simulink model "slm_paper"  (Simulink 8.6)
settings: Solver=ode45  StartTime=0.0  StopTime=30  RelTol=1e-3
libraries: mblibv1 x12, simulink x3, aerolibconvert2 x2
settings Model: Creator=debraj  LastModifiedBy=Ayansengupta17
settings SolverCC: ZeroCrossControl=DisableAll
settings DebuggingCC: FcnCallInpInsideContextMsg=UseLocalSettings
settings ConfigComp: CovSFcnEnable=off
settings SimMechanicsCC: VisOnUpdateDiagram=on  VisDuringSimulation=on
settings ConfigurationSet: Description=SimMechanics 2G

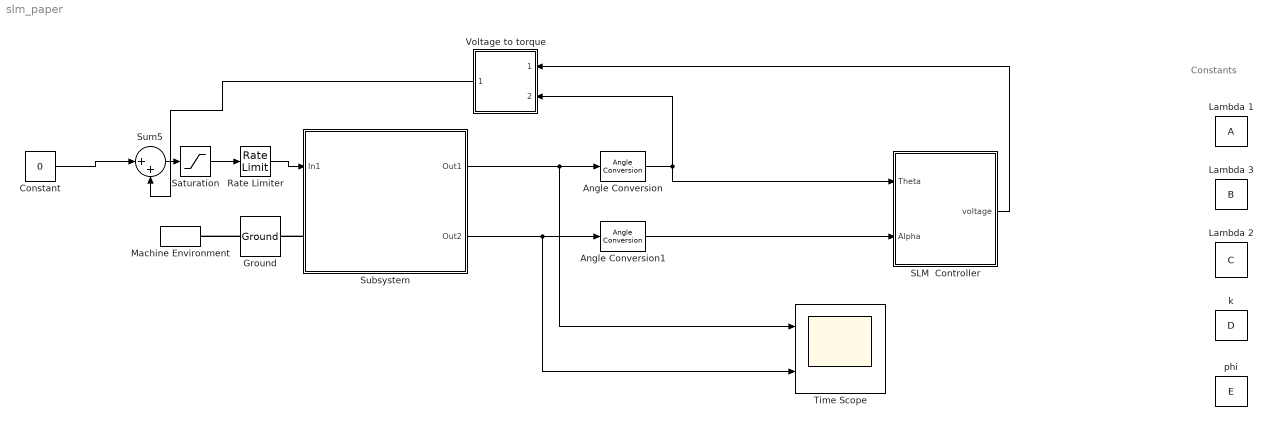
== system slm_paper ==
  note: Constants
  Angle Conversion : aerolibconvert2/Angle Conversion  IU=deg  OU=rad
  Angle Conversion1 : aerolibconvert2/Angle Conversion  IU=deg  OU=rad
  Constant : Constant  Value=0
  Ground : mblibv1/Bodies/Ground  UpdateFromCAD=off  LeftPortType=env  RightPortType=workingframe  PhysicalDomain=Mechanical  DialogClass=GroundBlock  CoordPosition=[0 0 0]  CoordPositionUnits=m  StateVectorMgrId=0  MachineId=[1 0]  ShowEnvPort=on  ParameterChecksum=[2459669987, 3834972678, 64255769, 951891124]  TopologyChecksum=[3132375730, 187115475, 220121263, 2848747769]
  Lambda 1 : DataStoreMemory  ReadBeforeWriteMsg=warning  WriteAfterWriteMsg=warning  WriteAfterReadMsg=warning  InitialValue=0.2
  Lambda 2 : DataStoreMemory  DataStoreName=C  ReadBeforeWriteMsg=warning  WriteAfterWriteMsg=warning  WriteAfterReadMsg=warning  InitialValue=0.9
  Lambda 3 : DataStoreMemory  DataStoreName=B  ReadBeforeWriteMsg=warning  WriteAfterWriteMsg=warning  WriteAfterReadMsg=warning  InitialValue=1
  Machine Environment : mblibv1/Bodies/Machine Environment  Tag=Factory ground  PortType=env  PhysicalDomain=Mechanical  DialogTemplateClass=MECH.MachineEnvironment  SyncWhenCopied=off  Gravity=[0 0 -9.81]  GravityUnits=m/s^2  GravityAsSignal=off  Dimensionality=Auto-detect  AnalysisType=Forward dynamics  LinearAssemblyTolerance=1e-3  LinearAssemblyToleranceUnits=m  AngularAssemblyTolerance=1e-3  AngularAssemblyToleranceUnits=rad  ConstraintSolverType=Stabilizing  ConstraintRelTolerance=1e-4  ConstraintAbsTolerance=1e-4  UseRobustSingularityHandling=off  RedundancyAnalysisToleranceType=Automatically select tolerance  RedundancyAnalysisTolerance=1e-14  StatePerturbationType=Fixed  PerturbationSize=1e-5  VisualizeMachine=on  BodyVisualizationType=Use model default body geometries  BodyColorSelMode=Use model default  DefaultBodyColor=[1 0 0]
  Rate Limiter : RateLimiter
  SLM  Controller : Subsystem
  Saturation : Saturate  UpperLimit=200  LowerLimit=-200  ZeroCross=off
  Subsystem : Subsystem
      mask init:
      | throttle = imread('spe_mech_invpend.jpg');
      mask Display: image(throttle)
  Sum5 : Sum  Inputs=|++
  Time Scope : Scope  NumInputPorts=2
  "Voltage to torque " : Subsystem
  k : DataStoreMemory  DataStoreName=D  ReadBeforeWriteMsg=warning  WriteAfterWriteMsg=warning  WriteAfterReadMsg=warning  InitialValue=9
  phi : DataStoreMemory  DataStoreName=E  ReadBeforeWriteMsg=warning  WriteAfterWriteMsg=warning  WriteAfterReadMsg=warning  InitialValue=0.5
  wires:
  Subsystem/2(Out2) -> Time Scope/2, Angle Conversion1/1
  Saturation/1 -> Rate Limiter/1
  Rate Limiter/1 -> Subsystem/1(In1)
  Sum5/1 -> Saturation/1
  Constant/1 -> Sum5/1
  Subsystem/1(Out1) -> Time Scope/1, Angle Conversion/1
  Angle Conversion/1 -> SLM  Controller/1(Theta), "Voltage to torque "/2(Theta)
  "Voltage to torque "/1("Torque ") -> Sum5/2
  Angle Conversion1/1 -> SLM  Controller/2("Alpha ")
  SLM  Controller/1("voltage ") -> "Voltage to torque "/1(voltage)
  connections:
  Ground/LConn1 -- Machine Environment/RConn1
  Subsystem/LConn1 -- Ground/RConn1

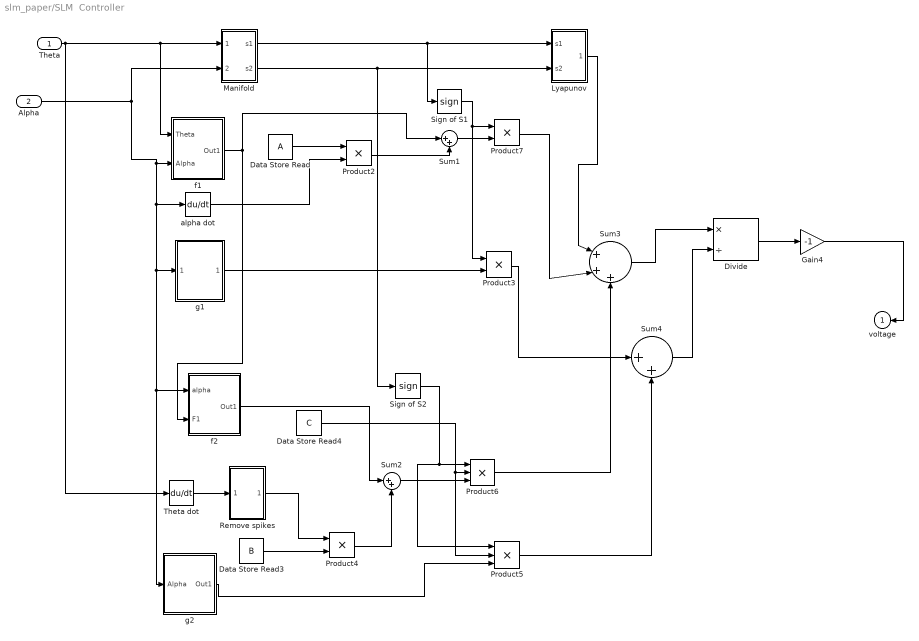
== system slm_paper/SLM  Controller ==
  Theta : Inport
  "Alpha " : Inport  Port=2
  Data Store Read : DataStoreRead
  Data Store Read3 : DataStoreRead  DataStoreName=B
  Data Store Read4 : DataStoreRead  DataStoreName=C
  Divide : Product  Inputs=*/
  Gain4 : Gain  Gain=-1
  "Lyapunov " : Subsystem
  Manifold : Subsystem
  Product{2..4,7} (4 alike) : Product
  Product5 : Product  Inputs=3
  Product6 : Product  Inputs=3
  Remove spikes : Subsystem
  Sign of S1 : Signum  ZeroCross=off
  Sign of S2 : Signum  ZeroCross=off
  Sum1 : Sum  Inputs=|++
  Sum2 : Sum  Inputs=|++
  Sum3 : Sum  Inputs=|+++
  Sum4 : Sum  Inputs=|++
  Theta dot : Derivative
  "alpha dot " : Derivative  CoefficientInTFapproximation=0.00001
  f1 : Subsystem
  f2 : Subsystem
  g1 : Subsystem
  g2 : Subsystem
  "voltage " : Outport
  wires:
  Product2/1 -> Sum1/2
  Sign of S1/1 -> Product3/1, Product7/1
  Sum1/1 -> Product7/2
  Sign of S2/1 -> Product6/1, Product5/1
  Sum2/1 -> Product6/3
  Product3/1 -> Sum4/1
  Manifold/1(s1) -> Sign of S1/1, "Lyapunov "/1(s1)
  Divide/1 -> Gain4/1
  Theta dot/1 -> Remove spikes/1(In1)
  "Lyapunov "/1(Out1) -> Sum3/1
  f2/1(Out1) -> Sum2/1
  Product5/1 -> Sum4/2
  Product4/1 -> Sum2/2
  Sum3/1 -> Divide/1
  Manifold/2(s2) -> Sign of S2/1, "Lyapunov "/2(s2)
  f1/1(Out1) -> Sum1/1, f2/2("F1 ")
  Sum4/1 -> Divide/2
  g2/1(Out1) -> Product5/3
  Data Store Read4/1 -> Product5/2, Product6/2
  Product7/1 -> Sum3/2
  Product6/1 -> Sum3/3
  "alpha dot "/1 -> Product2/2
  "Alpha "/1 -> Manifold/2("alpha "), "alpha dot "/1, f2/1(alpha), g2/1("Alpha "), g1/1("Alpha "), f1/2("Alpha ")
  Remove spikes/1(Out1) -> Product4/1
  Data Store Read3/1 -> Product4/2
  Gain4/1 -> "voltage "/1
  g1/1(Out1) -> Product3/2
  Data Store Read/1 -> Product2/1
  Theta/1 -> Theta dot/1, Manifold/1(theta), f1/1(Theta)

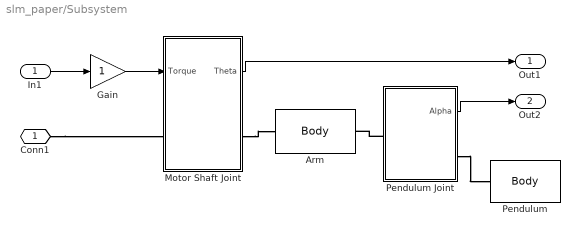
== system slm_paper/Subsystem ==
  In1 : Inport
  Arm : mblibv1/Bodies/Body  Tag=Factory generic  Description=Mechanical Blockset  LConnTagsString=CS1  RConnTagsString=CS2  UpdateFromCAD=off  DialogClass=MechanicalBodyBlock  Mass=0.028  MassUnits=kg  InertiaUnits=kg*m^2  Inertia=[0 0 0;0 0 0;0 0 0.000123]  Shape=Cylinder  ShapeDims=[1 1]  ShapeUnits=m  ShapeUse=false  Density=1  DensityUnits=kg/m^3  DensityUse=false  GraphicsMode=MACHINE_DEFAULT  BodyColorSelMode=MACHINE_DEFAULT  BodyColor=[1 0 0]  AttachedToCS=CG  CG=Left$CG$[0 0.08260/2 0]$CS1$CS1$m$[0 0 0]$Euler X-Y-Z$deg$WORLD$false$none  WorkingFrames=Left$CS1$[0 0 0]$WORLD$WORLD$m$[0 0 0]$Euler X-Y-Z$deg$WORLD$true$none#Right$CS2$[0 0.08260 0]$CS1$CS1$m$[0 0 0]$Euler X-Y-Z$deg$WORLD$true$none  CGPos=[0 0.08260/2 0]  CGRot=[0 0 0]  CS0Pos=[]  CS0Rot=[]  CS1Pos=[0 0 0]  CS1Rot=[0 0 0]  CS2Pos=[0 0.08260 0]  CS2Rot=[0 0 0]  CS3Pos=[]  CS3Rot=[]  CS4Pos=[]  CS4Rot=[]  CS5Pos=[]  CS5Rot=[]  CS6Pos=[]  CS6Rot=[]  CS7Pos=[]  CS7Rot=[]  CS8Pos=[]  CS8Rot=[]  CS9Pos=[]  CS9Rot=[]  CS10Pos=[]  CS10Rot=[]  CS11Pos=[]  CS11Rot=[]  CS12Pos=[]  CS12Rot=[]  CS13Pos=[]  CS13Rot=[]  CS14Pos=[]  CS14Rot=[]  CS15Pos=[]  CS15Rot=[]  CS16Pos=[]  CS16Rot=[]  CS17Pos=[]  CS17Rot=[]  CS18Pos=[]  CS18Rot=[]  CS19Pos=[]  CS19Rot=[]  CS20Pos=[]  CS20Rot=[]
  Gain : Gain
  Motor Shaft Joint : Subsystem
  Pendulum : mblibv1/Bodies/Body  Tag=Factory generic  Description=Mechanical Blockset  LConnTagsString=CS1  UpdateFromCAD=off  DialogClass=MechanicalBodyBlock  Mass=0.027  MassUnits=kg  InertiaUnits=kg*m^2  Inertia=[0 0 0;0 0 0;0 0 0.00011]  Shape=Cylinder  ShapeDims=[1 1]  ShapeUnits=m  ShapeUse=false  Density=1  DensityUnits=kg/m^3  DensityUse=false  GraphicsMode=MACHINE_DEFAULT  BodyColorSelMode=MACHINE_DEFAULT  BodyColor=[1 0 0]  AttachedToCS=CG  CG=Left$CG$[0 0 0.191/2]$CS1$CS1$m$[0 0 0]$Euler X-Y-Z$deg$WORLD$false$none  WorkingFrames=Left$CS1$[0 0 0]$ADJOINING$ADJOINING$m$[0 0 0]$Euler X-Y-Z$deg$WORLD$true$none#Right$CS2$[0 0 0.191]$CS1$CS1$m$[0 0 0]$Euler X-Y-Z$deg$WORLD$false$none  CGPos=[0 0 0.191/2]  CGRot=[0 0 0]  CS0Pos=[]  CS0Rot=[]  CS1Pos=[0 0 0]  CS1Rot=[0 0 0]  CS2Pos=[0 0 0.191]  CS2Rot=[0 0 0]  CS3Pos=[]  CS3Rot=[]  CS4Pos=[]  CS4Rot=[]  CS5Pos=[]  CS5Rot=[]  CS6Pos=[]  CS6Rot=[]  CS7Pos=[]  CS7Rot=[]  CS8Pos=[]  CS8Rot=[]  CS9Pos=[]  CS9Rot=[]  CS10Pos=[]  CS10Rot=[]  CS11Pos=[]  CS11Rot=[]  CS12Pos=[]  CS12Rot=[]  CS13Pos=[]  CS13Rot=[]  CS14Pos=[]  CS14Rot=[]  CS15Pos=[]  CS15Rot=[]  CS16Pos=[]  CS16Rot=[]  CS17Pos=[]  CS17Rot=[]  CS18Pos=[]  CS18Rot=[]  CS19Pos=[]  CS19Rot=[]  CS20Pos=[]  CS20Rot=[]
  Pendulum Joint : Subsystem
  Conn1 : PMIOPort  Port=1  Side=Left
  Out1 : Outport
  Out2 : Outport  Port=2
  wires:
  Motor Shaft Joint/1(Theta) -> Out1/1
  In1/1 -> Gain/1
  Pendulum Joint/1(Alpha) -> Out2/1
  Gain/1 -> Motor Shaft Joint/1(Torque)
  connections:
  Motor Shaft Joint/RConn1 -- Arm/LConn1
  Pendulum Joint/LConn1 -- Arm/RConn1
  Pendulum Joint/RConn1 -- Pendulum/LConn1
  Conn1/RConn1 -- Motor Shaft Joint/LConn1

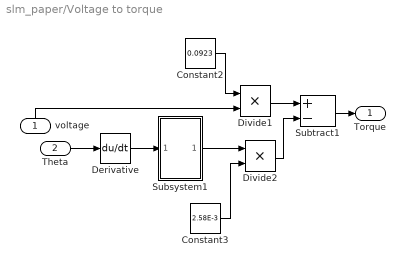
== system slm_paper/Voltage to torque  ==
  voltage : Inport
  Theta : Inport  Port=2
  Constant2 : Constant  Value=0.0923
  Constant3 : Constant  Value=2.58E-3
  Derivative : Derivative  CoefficientInTFapproximation=0.00001
  Divide1 : Product  Inputs=**
  Divide2 : Product  Inputs=**
  Subsystem1 : Subsystem
  Subtract1 : Sum  Inputs=+-
  "Torque " : Outport
  wires:
  Constant2/1 -> Divide1/1
  Subtract1/1 -> "Torque "/1
  Divide2/1 -> Subtract1/2
  Divide1/1 -> Subtract1/1
  voltage/1 -> Divide1/2
  Constant3/1 -> Divide2/2
  Theta/1 -> Derivative/1
  Derivative/1 -> Subsystem1/1(In1)
  Subsystem1/1(Out1) -> Divide2/1

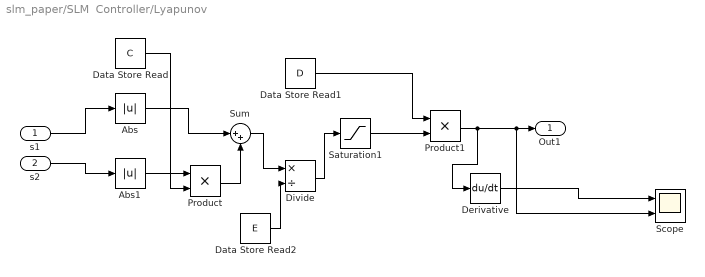
== system slm_paper/SLM  Controller/Lyapunov  ==
  s1 : Inport
  s2 : Inport  Port=2
  Abs : Abs
  Abs1 : Abs
  Data Store Read : DataStoreRead  DataStoreName=C
  Data Store Read1 : DataStoreRead  DataStoreName=D
  Data Store Read2 : DataStoreRead  DataStoreName=E
  Derivative : Derivative
  Divide : Product  Inputs=*/
  Product : Product
  Product1 : Product
  Saturation1 : Saturate  UpperLimit=1  LowerLimit=-1  ZeroCross=off
  Scope : Scope  NumInputPorts=2
  Sum : Sum  Inputs=|++
  Out1 : Outport
  wires:
  Data Store Read/1 -> Product/2
  s2/1 -> Abs1/1
  s1/1 -> Abs/1
  Abs1/1 -> Product/1
  Abs/1 -> Sum/1
  Product/1 -> Sum/2
  Saturation1/1 -> Product1/2
  Data Store Read1/1 -> Product1/1
  Sum/1 -> Divide/1
  Divide/1 -> Saturation1/1
  Data Store Read2/1 -> Divide/2
  Product1/1 -> Derivative/1, Scope/2, Out1/1
  Derivative/1 -> Scope/1

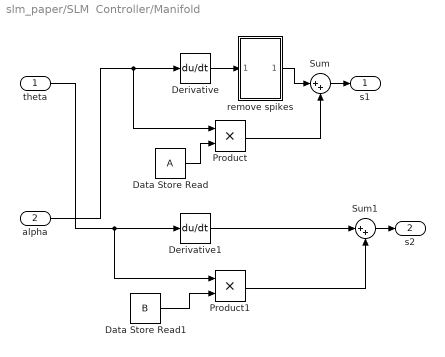
== system slm_paper/SLM  Controller/Manifold ==
  theta : Inport
  "alpha " : Inport  Port=2
  Data Store Read : DataStoreRead
  Data Store Read1 : DataStoreRead  DataStoreName=B
  Derivative : Derivative
  Derivative1 : Derivative
  Product : Product
  Product1 : Product
  Sum : Sum  Inputs=|++
  Sum1 : Sum  Inputs=|++
  "remove spikes " : Subsystem
  s1 : Outport
  s2 : Outport  Port=2
  wires:
  Sum/1 -> s1/1
  Sum1/1 -> s2/1
  Product/1 -> Sum/2
  Product1/1 -> Sum1/2
  Data Store Read/1 -> Product/2
  Data Store Read1/1 -> Product1/2
  Derivative1/1 -> Sum1/1
  Derivative/1 -> "remove spikes "/1(In1)
  "remove spikes "/1(Out1) -> Sum/1
  "alpha "/1 -> Product/1, Derivative/1
  theta/1 -> Product1/1, Derivative1/1

== system slm_paper/SLM  Controller/Remove spikes ==
  In1 : Inport
  Compare To Constant : simulink/Logic and Bit Operations/Compare To Constant  relop=<=  const=50  OutDataTypeStr=boolean
  Product1 : Product
  Out1 : Outport
  wires:
  In1/1 -> Product1/2, Compare To Constant/1
  Product1/1 -> Out1/1
  Compare To Constant/1 -> Product1/1

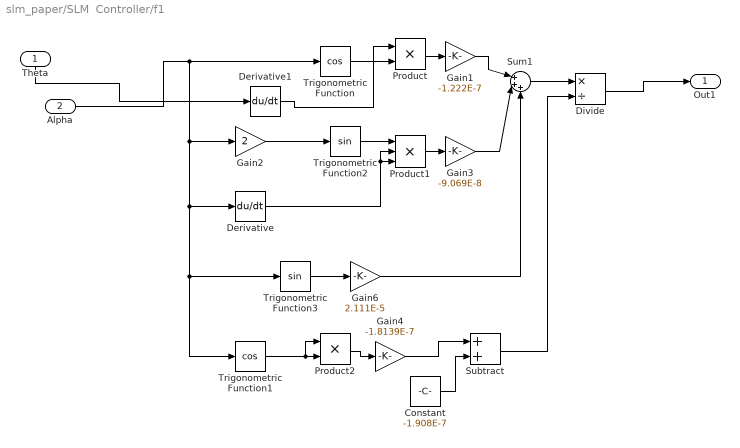
== system slm_paper/SLM  Controller/f1 ==
  Theta : Inport
  "Alpha " : Inport  Port=2
  Constant : Constant  Value=-1.908E-7
  Derivative : Derivative
  Derivative1 : Derivative
  Divide : Product  Inputs=*/
  Gain1 : Gain  Gain=-1.222E-7
  Gain2 : Gain  Gain=2
  Gain3 : Gain  Gain=-9.069E-8
  Gain4 : Gain  Gain=-1.8139E-7
  Gain6 : Gain  Gain=2.111E-5
  Product : Product
  Product1 : Product  Inputs=3
  Product2 : Product
  Subtract : Sum
  Sum1 : Sum  Inputs=|+++
  Trigonometric Function : Trigonometry  Operator=cos
  Trigonometric Function1 : Trigonometry  Operator=cos
  Trigonometric Function2 : Trigonometry
  Trigonometric Function3 : Trigonometry
  Out1 : Outport
  wires:
  Gain3/1 -> Sum1/2
  Trigonometric Function2/1 -> Product1/1
  Gain1/1 -> Sum1/1
  Trigonometric Function/1 -> Product/2
  Product1/1 -> Gain3/1
  Gain2/1 -> Trigonometric Function2/1
  Product/1 -> Gain1/1
  Trigonometric Function1/1 -> Product2/1, Product2/2
  Product2/1 -> Gain4/1
  Gain4/1 -> Subtract/1
  Constant/1 -> Subtract/2
  Sum1/1 -> Divide/1
  Subtract/1 -> Divide/2
  Divide/1 -> Out1/1
  Derivative/1 -> Product1/3, Product1/2
  Derivative1/1 -> Product/1
  Trigonometric Function3/1 -> Gain6/1
  Gain6/1 -> Sum1/3
  "Alpha "/1 -> Trigonometric Function3/1, Trigonometric Function1/1, Derivative/1, Gain2/1, Trigonometric Function/1
  Theta/1 -> Derivative1/1

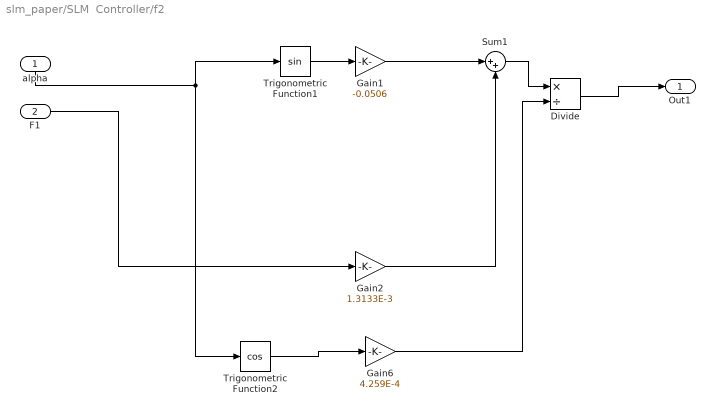
== system slm_paper/SLM  Controller/f2 ==
  alpha : Inport
  "F1 " : Inport  Port=2
  Divide : Product  Inputs=*/
  Gain1 : Gain  Gain=-0.0506
  Gain2 : Gain  Gain=1.3133E-3
  Gain6 : Gain  Gain=4.259E-4
  Sum1 : Sum  Inputs=|++
  Trigonometric Function1 : Trigonometry
  Trigonometric Function2 : Trigonometry  Operator=cos
  Out1 : Outport
  wires:
  "F1 "/1 -> Gain2/1
  alpha/1 -> Trigonometric Function1/1, Trigonometric Function2/1
  Sum1/1 -> Divide/1
  Divide/1 -> Out1/1
  Trigonometric Function2/1 -> Gain6/1
  Gain6/1 -> Divide/2
  Trigonometric Function1/1 -> Gain1/1
  Gain1/1 -> Sum1/1
  Gain2/1 -> Sum1/2

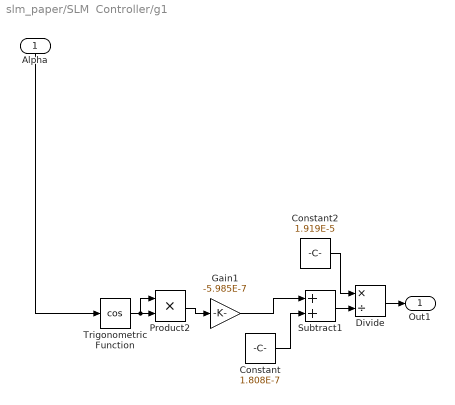
== system slm_paper/SLM  Controller/g1 ==
  "Alpha " : Inport
  Constant : Constant  Value=1.808E-7
  Constant2 : Constant  Value=1.919E-5
  Divide : Product  Inputs=*/
  Gain1 : Gain  Gain=-5.985E-7
  Product2 : Product
  Subtract1 : Sum
  Trigonometric Function : Trigonometry  Operator=cos
  Out1 : Outport
  wires:
  Subtract1/1 -> Divide/2
  Trigonometric Function/1 -> Product2/1, Product2/2
  Product2/1 -> Gain1/1
  Constant2/1 -> Divide/1
  "Alpha "/1 -> Trigonometric Function/1
  Divide/1 -> Out1/1
  Gain1/1 -> Subtract1/1
  Constant/1 -> Subtract1/2

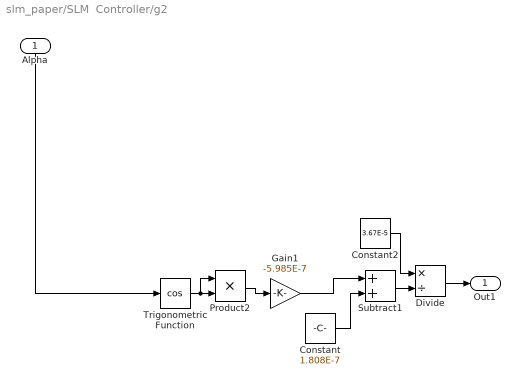
== system slm_paper/SLM  Controller/g2 ==
  "Alpha " : Inport
  Constant : Constant  Value=1.808E-7
  Constant2 : Constant  Value=3.67E-5
  Divide : Product  Inputs=*/
  Gain1 : Gain  Gain=-5.985E-7
  Product2 : Product
  Subtract1 : Sum
  Trigonometric Function : Trigonometry  Operator=cos
  Out1 : Outport
  wires:
  "Alpha "/1 -> Trigonometric Function/1
  Divide/1 -> Out1/1
  Subtract1/1 -> Divide/2
  Trigonometric Function/1 -> Product2/1, Product2/2
  Product2/1 -> Gain1/1
  Constant2/1 -> Divide/1
  Gain1/1 -> Subtract1/1
  Constant/1 -> Subtract1/2

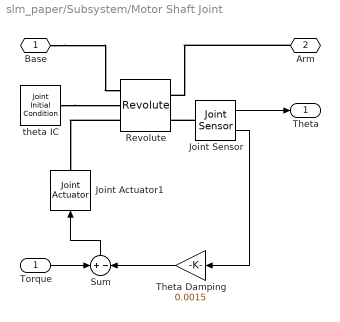
== system slm_paper/Subsystem/Motor Shaft Joint ==
  Torque : Inport
  Joint Actuator1 : mblibv1/Sensors &  Actuators/Joint Actuator  UpdateFromCAD=off  PhysicalDomain=Mechanical  PortType=blob  ActuationStyle=Force  AngleUnits=deg  ArcVelocityUnits=deg/s  ArcAccelerationUnits=deg/s^2  CoordPositionUnits=m  VelocityUnits=m/s  AccelerationUnits=m/s^2  ForceUnits=N  TorqueUnits=N-m  ActiveIO=on  Width=1  DialogClass=MechanicalActuatorBlock  Primitive=R1  ReferenceFrame=Absolute (World)
  Joint Sensor : mblibv1/Sensors &  Actuators/Joint Sensor  Description=Mechanical Blockset  UpdateFromCAD=off  PhysicalDomain=Mechanical  PortType=blob  Muxed=off  Pose=off  Angle=on  AngleUnits=deg  ArcVelocity=on  ArcVelocityUnits=rad/s  ArcAcceleration=off  ArcAccelerationUnits=deg/s^2  CoordPosition=on  CoordPositionUnits=m  Velocity=off  VelocityUnits=m/s  Acceleration=off  AccelerationUnits=m/s^2  Quaternion=on  QuaternionDT=off  QuaternionDDT=off  QuaternionUnits=off  OutputVector=[ 1 1 ]  ActiveIO=on  Width=2  DialogClass=MechanicalSensorBlock  Primitive=R1  Force=off  ForceUnits=N  Torque=off  TorqueUnits=N*m  ReferenceFrame=Absolute (INERTIAL)  ReactionSensedSide=Base  ReactionReferenceFrame=Absolute (World)  ReactionForce=off  ReactionForceUnits=N  ReactionMoment=off  ReactionMomentUnits=N*m
  Revolute : mblibv1/Joints/Revolute  Tag=Factory generic  Description=Mechanical Blockset  LConnTagsString=__newl0|SA1|SA2  RConnTagsString=__newr0|SA1  UpdateFromCAD=off  NumSAPorts=3  CutJoint=off  MarkAsCut=off  Primitives=revolute  PrimitiveProps=R1$Base$[0 0 1]$revolute  DialogClass=JointBlock  R1Axis=[0 0 1]
  Sum : Sum  Inputs=+|-  SaturateOnIntegerOverflow=on  InputSameDT=on  OutDataTypeStr=Inherit: Same as first input
  Theta Damping : Gain  Gain=0.0015  SaturateOnIntegerOverflow=on  OutDataTypeStr=Inherit: Same as input  ParamDataTypeStr=Inherit: Same as input
  theta IC : mblibv1/Sensors &  Actuators/Joint Initial Condition  Description=Mechanical Blockset  UpdateFromCAD=off  LeftPortType=blob  RightPortType=blob  PhysicalDomain=Mechanical  DialogClass=InitialConditionBlock  Primitive=R1  CoordPosition=0  Velocity=0.0  AngleUnits=deg  ArcVelocityUnits=deg/s  CoordPositionUnits=m  VelocityUnits=m/s  InitialConditions=P1$false$0$m$rad$0$m/s$rad/s#P2$false$0$m$rad$0$m/s$rad/s#P3$false$0$m$rad$0$m/s$rad/s#R1$true$0$m$deg$0.0$m/s$deg/s#R2$false$0$m$rad$0$m/s$rad/s#R3$false$0$m$rad$0$m/s$rad/s#S$false$0$m$rad$0$m/s$rad/s  P1PIC=0  P1VIC=0  P2PIC=0  P2VIC=0  P3PIC=0  P3VIC=0  R1PIC=0  R1VIC=0.0  R2PIC=0  R2VIC=0  R3PIC=0  R3VIC=0  SPIC=0  SVIC=0
  Base : PMIOPort  Port=1  Side=Left
  Arm : PMIOPort  Port=2  Side=Right
  Theta : Outport
  wires:
  Joint Sensor/2 -> Theta Damping/1
  Joint Sensor/1 -> Theta/1
  Torque/1 -> Sum/1
  Theta Damping/1 -> Sum/2
  Sum/1 -> Joint Actuator1/1
  connections:
  Joint Sensor/LConn1 -- Revolute/RConn2
  Revolute/LConn3 -- Joint Actuator1/RConn1
  theta IC/RConn1 -- Revolute/LConn2
  Arm/RConn1 -- Revolute/RConn1
  Base/RConn1 -- Revolute/LConn1

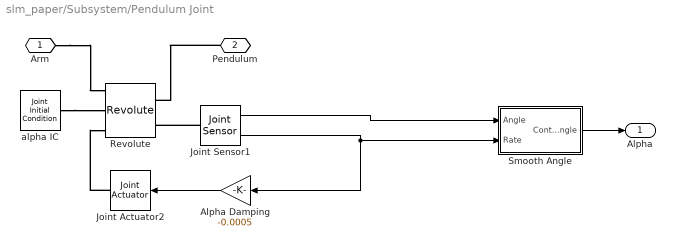
== system slm_paper/Subsystem/Pendulum Joint ==
  Alpha Damping : Gain  Gain=-0.0005  SaturateOnIntegerOverflow=on  OutDataTypeStr=Inherit: Same as input  ParamDataTypeStr=Inherit: Same as input
  Joint Actuator2 : mblibv1/Sensors &  Actuators/Joint Actuator  Description=Mechanical Blockset  UpdateFromCAD=off  PhysicalDomain=Mechanical  PortType=blob  ActuationStyle=Force  AngleUnits=deg  ArcVelocityUnits=deg/s  ArcAccelerationUnits=deg/s^2  CoordPositionUnits=m  VelocityUnits=m/s  AccelerationUnits=m/s^2  ForceUnits=N  TorqueUnits=N-m  ActiveIO=on  Width=1  DialogClass=MechanicalActuatorBlock  Primitive=R1  ReferenceFrame=Absolute (INERTIAL)
  Joint Sensor1 : mblibv1/Sensors &  Actuators/Joint Sensor  Description=Mechanical Blockset  UpdateFromCAD=off  PhysicalDomain=Mechanical  PortType=blob  Muxed=off  Pose=off  Angle=on  AngleUnits=deg  ArcVelocity=on  ArcVelocityUnits=rad/s  ArcAcceleration=off  ArcAccelerationUnits=deg/s^2  CoordPosition=on  CoordPositionUnits=m  Velocity=off  VelocityUnits=m/s  Acceleration=off  AccelerationUnits=m/s^2  Quaternion=on  QuaternionDT=off  QuaternionDDT=off  QuaternionUnits=off  OutputVector=[ 1 1 ]  ActiveIO=on  Width=2  DialogClass=MechanicalSensorBlock  Primitive=R1  Force=off  ForceUnits=N  Torque=off  TorqueUnits=N*m  ReferenceFrame=Absolute (INERTIAL)  ReactionSensedSide=Base  ReactionReferenceFrame=Absolute (World)  ReactionForce=off  ReactionForceUnits=N  ReactionMoment=off  ReactionMomentUnits=N*m
  Revolute : mblibv1/Joints/Revolute  Tag=Factory generic  Description=Mechanical Blockset  LConnTagsString=__newl0|SA1|SA2  RConnTagsString=__newr0|SA1  UpdateFromCAD=off  NumSAPorts=3  CutJoint=off  MarkAsCut=off  Primitives=revolute  PrimitiveProps=R1$Base$[0 1 0]$revolute  DialogClass=JointBlock  R1Axis=[0 1 0]
  Smooth Angle : Subsystem  mask{rad=deg, rads=rad/s}
      mask prompts: rad "Angle measured in:"; rads "Rate measured in:"
      mask help: Constructs continuous angle from angular velocity rate and piecewise continuous angle measured by Joint Sensor on a revolute primitive. Integrates angular velocity to determine number of revolutions that the joint primitive has undergone.
      mask TypeOptions rad: rad | deg
      mask TypeOptions rads: rad/s | deg/s
  alpha IC : mblibv1/Sensors &  Actuators/Joint Initial Condition  Description=Mechanical Blockset  UpdateFromCAD=off  LeftPortType=blob  RightPortType=blob  PhysicalDomain=Mechanical  DialogClass=InitialConditionBlock  Primitive=R1  CoordPosition=10  Velocity=0.0  AngleUnits=deg  ArcVelocityUnits=deg/s  CoordPositionUnits=m  VelocityUnits=m/s  InitialConditions=P1$false$0$m$rad$0$m/s$rad/s#P2$false$0$m$rad$0$m/s$rad/s#P3$false$0$m$rad$0$m/s$rad/s#R1$true$10$m$deg$0.0$m/s$deg/s#R2$false$0$m$rad$0$m/s$rad/s#R3$false$0$m$rad$0$m/s$rad/s#S$false$0$m$rad$0$m/s$rad/s  P1PIC=0  P1VIC=0  P2PIC=0  P2VIC=0  P3PIC=0  P3VIC=0  R1PIC=10  R1VIC=0.0  R2PIC=0  R2VIC=0  R3PIC=0  R3VIC=0  SPIC=0  SVIC=0
  Arm : PMIOPort  Port=1  Side=Left
  Pendulum : PMIOPort  Port=2  Side=Right
  Alpha : Outport
  wires:
  Joint Sensor1/1 -> Smooth Angle/1(Angle)
  Joint Sensor1/2 -> Alpha Damping/1, Smooth Angle/2(Rate)
  Alpha Damping/1 -> Joint Actuator2/1
  Smooth Angle/1(Continuous Angle) -> Alpha/1
  connections:
  Joint Sensor1/LConn1 -- Revolute/RConn2
  alpha IC/RConn1 -- Revolute/LConn2
  Joint Actuator2/RConn1 -- Revolute/LConn3
  Arm/RConn1 -- Revolute/LConn1
  Pendulum/RConn1 -- Revolute/RConn1

== system slm_paper/Voltage to torque /Subsystem1 ==
  In1 : Inport
  Compare To Constant : simulink/Logic and Bit Operations/Compare To Constant  relop=<=  const=50  OutDataTypeStr=boolean
  Product1 : Product
  Out1 : Outport
  wires:
  In1/1 -> Product1/2, Compare To Constant/1
  Product1/1 -> Out1/1
  Compare To Constant/1 -> Product1/1

== system slm_paper/SLM  Controller/Manifold/remove spikes  ==
  In1 : Inport
  Compare To Constant : simulink/Logic and Bit Operations/Compare To Constant  relop=<=  const=50  OutDataTypeStr=boolean
  Product1 : Product
  Out1 : Outport
  wires:
  In1/1 -> Product1/2, Compare To Constant/1
  Product1/1 -> Out1/1
  Compare To Constant/1 -> Product1/1

== system slm_paper/Subsystem/Pendulum Joint/Smooth Angle ==
  Angle : Inport
  Rate : Inport  Port=2
  Fcn1 : Fcn  Expr=u(2) + (2*(u(1) > u(2)) - 1)*2*pi*floor(abs(u(1)-u(2))/(2*pi) + 0.5)
  Gain1 : Gain  Gain=rad+(pi/180-2)*(rad-1)  SaturateOnIntegerOverflow=on  OutDataTypeStr=Inherit: Same as input  ParamDataTypeStr=Inherit: Same as input
  Gain3 : Gain  Gain=rads+(pi/180-2)*(rads-1)  SaturateOnIntegerOverflow=on  OutDataTypeStr=Inherit: Same as input  ParamDataTypeStr=Inherit: Same as input
  Gain4 : Gain  Gain=rad+(180/pi-2)*(rad-1)  SaturateOnIntegerOverflow=on  OutDataTypeStr=Inherit: Same as input  ParamDataTypeStr=Inherit: Same as input
  Integrator : Integrator  AbsoluteTolerance=1e-3
  Mux : Mux  Inputs=2
  Continuous Angle : Outport
  wires:
  Gain1/1 -> Mux/2
  Gain3/1 -> Integrator/1
  Integrator/1 -> Mux/1
  Mux/1 -> Fcn1/1
  Fcn1/1 -> Gain4/1
  Rate/1 -> Gain3/1
  Angle/1 -> Gain1/1
  Gain4/1 -> Continuous Angle/1
